simulink model "simple"  (Simulink 5.0)
settings: Solver=ode45  StartTime=t_init  StopTime=t_final  RelTol=1e-3
values from neighbouring files (symbols this model uses):
  B = zeros(1,degB+1)    [ext.m]
  C = [C Ck]    [polmul.m]
  D = D/D(1)    [tfvar.m]
undefined symbols (not defined in the file or in its folder): A, R, S, st, st1, Ts, zk
settings Model: Creator=kannan  LastModifiedBy=kannan  ExtModeAutoUpdateStatusClock=off

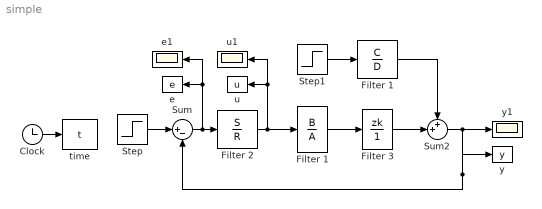
== system simple ==
  " Filter 1" : DiscreteFilter  Numerator=B  Denominator=A  SampleTime=Ts
  " Filter 2" : DiscreteFilter  Numerator=S  Denominator=R  SampleTime=Ts
  " Filter 3" : DiscreteFilter  Numerator=zk  Denominator=1  SampleTime=Ts
  Clock : Clock
      settings: Decimation=10
  Filter 1 : DiscreteFilter  Numerator=C  Denominator=D  SampleTime=Ts
  Step : Step  Time=0  After=st  SampleTime=Ts
  Step1 : Step  Time=0  After=st1  SampleTime=Ts
  Sum : Sum  Inputs=|+-  SaturateOnIntegerOverflow=on
  Sum2 : Sum  Inputs=++|  SaturateOnIntegerOverflow=on
  e : ToWorkspace  VariableName=e  SampleTime=Ts  SaveFormat=Array
  e1 : Scope
      settings: YMin=-6e+164  YMax=1.02293e+149  SaveName=ScopeData2
  time : ToWorkspace  VariableName=t  SampleTime=Ts  SaveFormat=Array
  u : ToWorkspace  VariableName=u  SampleTime=Ts  SaveFormat=Array
  u1 : Scope
      settings: YMin=-6e+164  YMax=1.02293e+149
  y : ToWorkspace  VariableName=y  SampleTime=Ts  SaveFormat=Array
  y1 : Scope
      settings: YMin=-6e+164  YMax=1.02293e+149
  wires:
  Clock/1 -> time/1
  Sum/1 -> " Filter 2"/1, e/1, e1/1
  " Filter 2"/1 -> u1/1, u/1, " Filter 1"/1
  " Filter 1"/1 -> " Filter 3"/1
  " Filter 3"/1 -> Sum2/2
  Sum2/1 -> y1/1, y/1, Sum/2
  Step1/1 -> Filter 1/1
  Filter 1/1 -> Sum2/1
  Step/1 -> Sum/1
